simulink model "PID_Controller"  (R2020b)
settings: Solver=ode4  StartTime=0.0  StopTime=30.399  FixedStep=1e-3  RelTol=1e-3
values from neighbouring files (symbols this model uses):
  H_I = SYS_I    [Draft_Parameter_Determining_Code.m]
  H_N = SYS_N    [Draft_Parameter_Determining_Code.m]
  Kd = 0.105 * Kcr * Pcr    [Draft_Parameter_Determining_Code.m]
  Ki = 1.75 * Kcr / Pcr    [Draft_Parameter_Determining_Code.m]
  Kp = 0.7 * Kcr    (= 0.0293125)    [Draft_Parameter_Determining_Code.m]
libraries: pid_lib x1
settings Model: Creator=chris  LastModifiedBy=chris

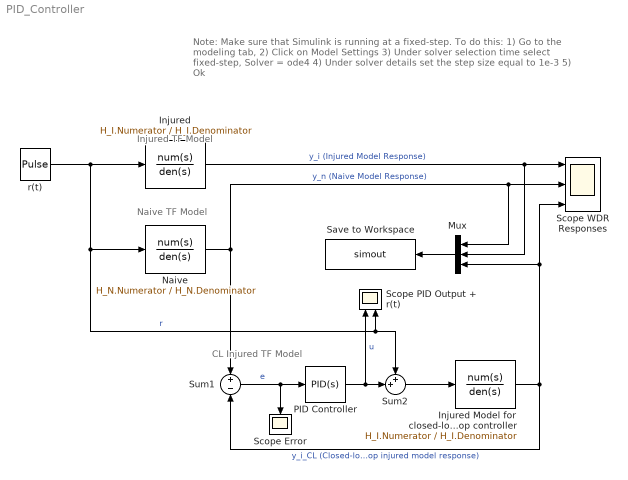
== system PID_Controller ==
  note: Injured TF Model
  note: Note: Make sure that Simulink is running at a fixed-step. To do this:
      | 1) Go to the modeling tab,
      | 2) Click on Model Settings
      | 3) Under solver selection time select fixed-step, Solver = ode4
      | 4) Under solver details set the step size equal to 1e-3
      | 5) Ok
  note: Naive TF Model
  note: CL Injured TF Model
  Injured : TransferFcn  Numerator=H_I.Numerator  Denominator=H_I.Denominator
  Injured Model for closed-loop controller : TransferFcn  Numerator=H_I.Numerator  Denominator=H_I.Denominator
  Mux : Mux  Inputs=3
  Naive : TransferFcn  Numerator=H_N.Numerator  Denominator=H_N.Denominator
  PID Controller : pid_lib/PID Controller  Controller=PID  Form=Parallel  TimeDomain=Continuous-time  UseExternalTs=off  SampleTime=-1  IntegratorMethod=Forward Euler  FilterMethod=Forward Euler  ControllerParametersSource=internal  P=Kp  I=Ki  D=Kd  UseFilter=on  N=1000  TunerSelectOption=Transfer Function Based (PID Tuner App)  InitialConditionSource=internal  InitialConditionForIntegrator=0  InitialConditionForFilter=0  DifferentiatorICPrevScaledInput=0  ExternalReset=none  TrackingMode=off  Kt=1  LimitOutput=off  SatLimitsSource=internal  UpperSaturationLimit=inf  LowerSaturationLimit=-inf  LinearizeAsGain=on  AntiWindupMode=none  Kb=1  POutMin=[]  POutMax=[]  IOutMin=[]  IOutMax=[]  DOutMin=[]  DOutMax=[]  NOutMin=[]  NOutMax=[]  SumOutMin=[]  SumOutMax=[]  SaturationOutMin=[]  SaturationOutMax=[]  PParamMin=[]  PParamMax=[]  IParamMin=[]  IParamMax=[]  DParamMin=[]  DParamMax=[]  NParamMin=[]  NParamMax=[]  KbParamMin=[]  KbParamMax=[]  KtParamMin=[]  KtParamMax=[]  KbOutMin=[]  KbOutMax=[]  KtOutMin=[]  KtOutMax=[]  IntegratorOutMin=[]  IntegratorOutMax=[]  FilterOutMin=[]  FilterOutMax=[]  SumI1OutMin=[]  SumI1OutMax=[]  SumI2OutMin=[]  SumI2OutMax=[]  SumI3OutMin=[]  SumI3OutMax=[]  SumI4OutMin=[]  SumI4OutMax=[]  SumDOutMin=[]  SumDOutMax=[]  DifferentiatorOutMin=[]  DifferentiatorOutMax=[]  FilterDiffOutCoefMin=[]  FilterDiffOutCoefMax=[]  ReciprocalOutMin=[]  ReciprocalOutMax=[]  SumDenOutMin=[]  SumDenOutMax=[]  SumNumOutMin=[]  SumNumOutMax=[]  DivideOutMin=[]  DivideOutMax=[]  UdiffTsProdOutMin=[]  UdiffTsProdOutMax=[]  NTsProdOutMin=[]  NTsProdOutMax=[]  UintegralTsProdOutMin=[]  UintegralTsProdOutMax=[]  UngainTsProdOutMin=[]  UngainTsProdOutMax=[]  IntegratorContinuousStateAttributes=''  IntegratorStateMustResolveToSignalObject=off  IntegratorRTWStateStorageClass=Auto  FilterContinuousStateAttributes=''  FilterStateMustResolveToSignalObject=off  FilterRTWStateStorageClass=Auto  ParallelPVariant=InternalParameters  IdealPVariant=Disabled  IVariant=InternalParameters  DVariant=InternalParameters  IntegratorVariant=Continuous  SatVariant=Disabled  AWVariant=Passthrough  PCopyVariant=Disabled  TRVariant=Disabled  FdbkBlocksVariant=Forward  IdealPFdbkVariant=Disabled  SatFdbkVariant=Disabled  DerivativeFilterVariant=ContFilter  NVariant=InternalParameters  NCopyVariant=Disabled  FilterICVariant=InternalICsFilter  IntegratorICVariant=InternalICs  ExternalResetVariant=Disabled  TRSumVariant=Passthrough  SumFdbkVariant=Disabled  SumVariant=Sum_PID  TsampFilterVariant=InternalTs  TsampNgainVariant=Passthrough  TsampIntegralVariant=Passthrough  ExternalSaturationOutDataTypeStr=Inherit: Same as second input
  Save to Workspace : ToWorkspace  VariableName=simout  SaveFormat=Structure With Time  SampleTime=-1
  Scope Error : Scope
  Scope PID Output + r(t) : Scope  NumInputPorts=2
  Scope WDR Responses : Scope  NumInputPorts=3
  Sum1 : Sum  Inputs=+|-
  Sum2 : Sum  Inputs=++|
  r(t) : DiscretePulseGenerator  PulseType=Time based  PulseWidth=.05  PhaseDelay=.001
  wires:
  r(t)/1 -> Injured/1, Naive/1, Sum2/1, Scope PID Output + r(t)/2  "r"
  Naive/1 -> Mux/1, Scope WDR Responses/2, Sum1/1  "y_n (Naive Model Response)"
  Sum1/1 -> PID Controller/1, Scope Error/1  "e"
  Injured/1 -> Mux/2, Scope WDR Responses/1  "y_i (Injured Model Response)"
  PID Controller/1 -> Sum2/2, Scope PID Output + r(t)/1  "u"
  Sum2/1 -> Injured Model for closed-loop controller/1
  Injured Model for closed-loop controller/1 -> Scope WDR Responses/3, Mux/3, Sum1/2  "y_i_CL (Closed-loop injured model response)"
  Mux/1 -> Save to Workspace/1
